simulink model "hour_meter_task"  (Simulink 3.00)
libraries: mathlib x9, analoglib x2, genlib x1

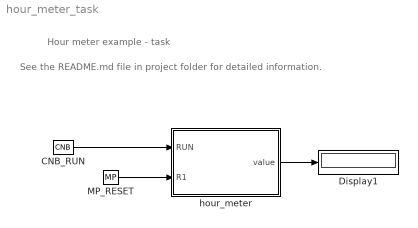
== system hour_meter_task ==
  note: See the README.md file in project folder for detailed information.
  note: Hour meter example - task
  CNB_RUN : mathlib/CNB  YCN=on
  Display1 : Display
      settings: Format=short
  MP_RESET : genlib/MP  BSTATE=off  pwidth=1  RPTF=off
  hour_meter : Subsystem  mask(REX sequence){unit=3: Hours}
      mask prompts: unit "Units of the hour meter"
      mask StyleString: popup(1: Seconds|2: Minutes|3: Hours|4: Days)
  wires:
  CNB_RUN/1 -> hour_meter/1(RUN)
  MP_RESET/1 -> hour_meter/2(R1)
  hour_meter/1(value) -> Display1/1

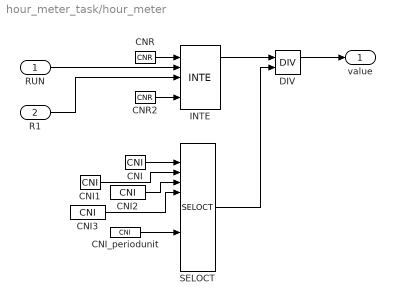
== system hour_meter_task/hour_meter ==
  RUN : Inport  Port=1
  R1 : Inport  Port=2
  CNI : mathlib/CNI  icn=1
  CNI1 : mathlib/CNI  icn=60
  CNI2 : mathlib/CNI  icn=3600
  CNI3 : mathlib/CNI  icn=86400
  CNI_periodunit : mathlib/CNI  icn=unit
  CNR : mathlib/CNR  ycn=1
  CNR2 : mathlib/CNR  ycn=1
  DIV : mathlib/DIV  yerr=1.0000000E+000
  INTE : analoglib/INTE  ymin=-1e300  ymax=1e300
  SELOCT : analoglib/SELOCT  BINF=off
  value : Outport  Port=1
  wires:
  CNI/1 -> SELOCT/2
  CNI1/1 -> SELOCT/3
  CNI2/1 -> SELOCT/4
  CNI3/1 -> SELOCT/5
  CNI_periodunit/1 -> SELOCT/9
  CNR/1 -> INTE/1
  CNR2/1 -> INTE/5
  DIV/1 -> value/1
  INTE/1 -> DIV/1
  R1/1 -> INTE/3
  RUN/1 -> INTE/2
  SELOCT/1 -> DIV/2
